simulink model "deconstructedpwm"  (R2020b)
settings: Solver=FixedStepAuto  StartTime=0.0  StopTime=1  FixedStep=1e-6  RelTol=1e-3
libraries: powerlib x11, simulink x3, powerlib_meascontrol x1
settings Model: Creator=adam_  LastModifiedBy=adam_

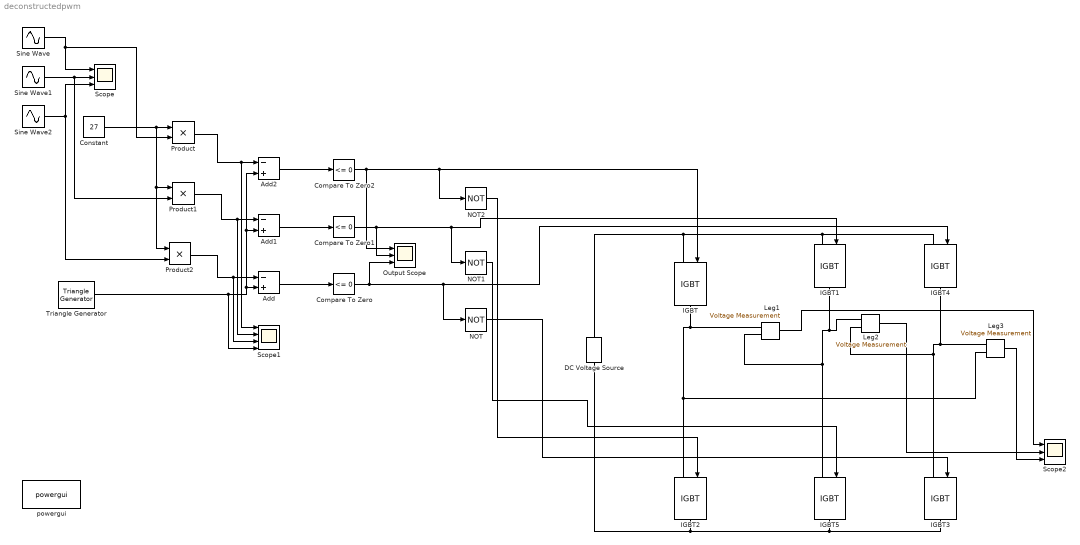
== system deconstructedpwm ==
  Add : Sum  Inputs=-+
  Add1 : Sum  Inputs=-+
  Add2 : Sum  Inputs=-+
  Compare To Zero : simulink/Logic and Bit Operations/Compare To Zero  relop=<=  OutDataTypeStr=boolean
  Compare To Zero1 : simulink/Logic and Bit Operations/Compare To Zero  relop=<=  OutDataTypeStr=boolean  ZeroCross=off
  Compare To Zero2 : simulink/Logic and Bit Operations/Compare To Zero  relop=<=  OutDataTypeStr=boolean
  Constant : Constant  Value=27
  DC Voltage Source : powerlib/Electrical Sources/DC Voltage Source  Amplitude=200  Measurements=None
  IGBT{,1..5} (6 alike) : powerlib/Power Electronics/IGBT  Ron=0.001  Lon=0  Vf=1  Tf=1e-6  Tt=2e-6  IC=0  Rs=1e5  Cs=inf  Measurements=off
  Leg1 : powerlib/Measurements/Voltage Measurement  PhasorSimulation=off  OutputType=Complex  PSBequivalent=0
  Leg2 : powerlib/Measurements/Voltage Measurement  PhasorSimulation=off  OutputType=Complex  PSBequivalent=0
  Leg3 : powerlib/Measurements/Voltage Measurement  PhasorSimulation=off  OutputType=Complex  PSBequivalent=0
  NOT : Logic  Operator=NOT  IconShape=distinctive  AllPortsSameDT=off  OutDataTypeStr=boolean
  NOT1 : Logic  Operator=NOT  IconShape=distinctive  AllPortsSameDT=off  OutDataTypeStr=boolean
  NOT2 : Logic  Operator=NOT  IconShape=distinctive  AllPortsSameDT=off  OutDataTypeStr=boolean
  Output Scope : Scope  NumInputPorts=3
  Product : Product
  Product1 : Product
  Product2 : Product
  Scope : Scope  NumInputPorts=3
  Scope1 : Scope  NumInputPorts=4
  Scope2 : Scope  NumInputPorts=3
  Sine Wave : Sin  Frequency=2*pi*60  SampleTime=0
  Sine Wave1 : Sin  Frequency=2*pi*60  Phase=2*pi/3  SampleTime=0
  Sine Wave2 : Sin  Frequency=2*pi*60  Phase=4*pi/3  SampleTime=0
  Triangle Generator : powerlib_meascontrol/Pulse & Signal Generators/Triangle Generator  Freq=1e3  Phase=90  Ts=1e-6
  powergui : powerlib/powergui  Priority=1  SimulationMode=Continuous  SampleTime=50e-6  frequency=60  Iterations=50  frequencyindice=0  Pbase=100e6  ErrMax=1e-4  UnitsV=kV  UnitsW=MW  buscounter=0  FunctionMessages=off  echomessages=off  EnableUseOfTLC=off  CurrentSourceSwitches=off  DisableSnubberDevices=off  DisableRonSwitches=off  DisableVfSwitches=off  DisplayEquations=off  AutomaticDiscreteSolvers=off  SolverType=Tustin/Backward Euler (TBE)  Interpol=off  ExternalGateDelay=off  methode=off  Ts=100  x0status=blocks  SPID=on  SwTol=0  HookPort=off  NonlinearTolerance=1e-4  nMaxIteration=100  ContinueOnMaxIteration=off  RestoreLinks=warning  ResistiveCurrentMeasurement=off  Frange=[0:2:500]  Ylog=off  Xlog=on  ShowGrid=off  save=off  variable=ZData  structure=0  ZoomFFT=off  StartTime=0.0  cycles=1  DisplayStyle=1  fundamental=60  FreqAxis=off  MaxFrequency=1000  frequencyindicesteady=1  RmsSteady=1  display=off
  wires:
  Sine Wave/1 -> Product/2, Scope/1
  Sine Wave1/1 -> Product1/2, Scope/2
  Sine Wave2/1 -> Scope/3, Product2/2
  Triangle Generator/1 -> Scope1/4, Add/2, Add2/2, Add1/2
  Product1/1 -> Scope1/2, Add1/1
  Add/1 -> Compare To Zero/1
  Add2/1 -> Compare To Zero2/1
  Product/1 -> Scope1/1, Add2/1
  Add1/1 -> Compare To Zero1/1
  Product2/1 -> Scope1/3, Add/1
  Constant/1 -> Product2/1, Product1/1, Product/1
  Leg2/1 -> Scope2/2
  NOT/1 -> IGBT3/1
  Leg1/1 -> Scope2/1
  Compare To Zero1/1 -> Output Scope/2, IGBT1/1, NOT1/1
  NOT2/1 -> IGBT2/1
  Compare To Zero2/1 -> IGBT/1, NOT2/1, Output Scope/1
  NOT1/1 -> IGBT5/1
  Leg3/1 -> Scope2/3
  Compare To Zero/1 -> IGBT4/1, NOT/1, Output Scope/3
  connections:
  IGBT4/RConn1 -- Leg3/LConn1 -- IGBT3/LConn1 -- Leg2/LConn2
  IGBT/LConn1 -- DC Voltage Source/RConn1 -- IGBT4/LConn1 -- IGBT1/LConn1
  IGBT2/RConn1 -- DC Voltage Source/LConn1 -- IGBT3/RConn1 -- IGBT5/RConn1
  IGBT5/LConn1 -- Leg1/LConn2 -- Leg2/LConn1 -- IGBT1/RConn1
  Leg3/LConn2 -- IGBT2/LConn1 -- IGBT/RConn1 -- Leg1/LConn1
